simulink model "FullED"  (R2023b)
settings: Solver=VariableStepAuto  StartTime=0.0  StopTime=3000/fs  RelTol=1e-3
undefined symbols (not defined in the file): exp_W1, exp_W2, exp_W3, exp_W4, fs
libraries: hdlBasic x155, hdlDSPIP x8, hdlsllib x2, vmcUtilities x1
(part 1 of 2)
settings Model: Creator=jojok  LastModifiedBy=jojok

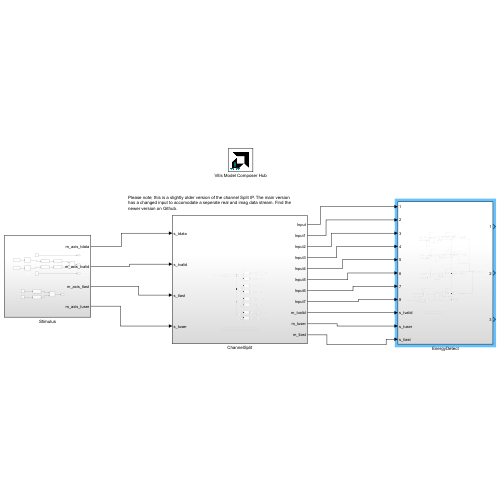
[thumbnail: Simulink's stored preview of the top-level diagram]
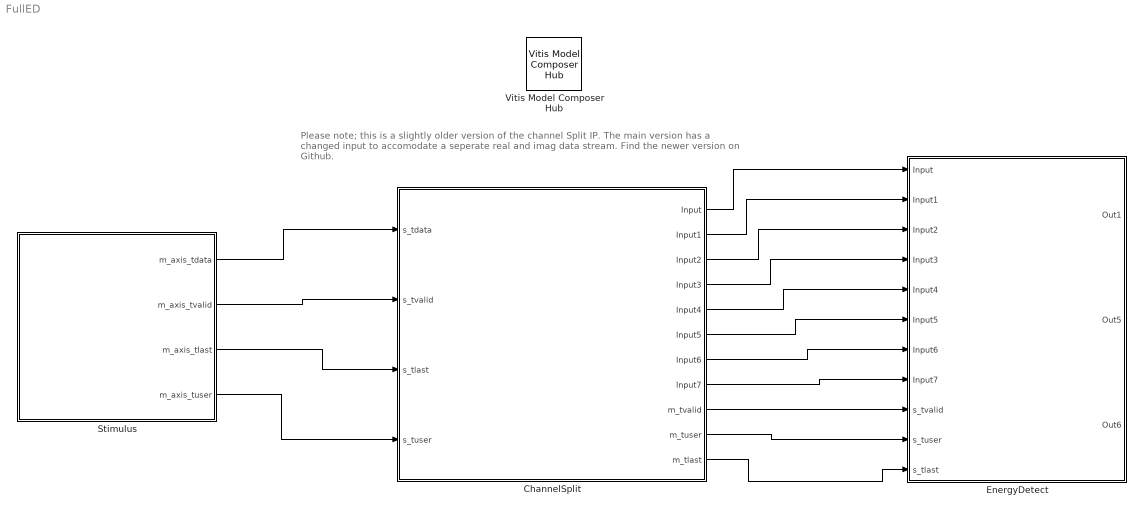
== system FullED ==
  note: Please note; this is a slightly older version of the channel Split IP. The main version
      | has a changed input to accomodate a seperate real and imag data stream. Find the newer version on Github.
  ChannelSplit : Subsystem
  EnergyDetect : Subsystem
  Stimulus : Subsystem
  Vitis Model Composer Hub : vmcUtilities/Vitis Model Composer Hub  Tag=genX  CodeGeneration=off  SubsystemName=ChannelSplit  DUTSubsystemName=EnergyDetect  CompilationType=HDLCompilation  ExportTypeV2=IP Catalog  TargetDirectory=./netlistFullED\ip\EnergyDetect\src  exportDesign=on  analyzeDesign=off  validateDesignOnHw=off  ExportType=HDL  IpVendor=xilinx.com  IpLibrary=hls  IpVersion=1.0  IpHWLanguage=Verilog  AieCompilerOptions={}  AieSimulatorOptions={}  CreateTestbench=off  TestbenchStackSize=10  RunRtlSim=off  RunCSim=off  RunAieSim=off  AieSimTimeout=50000  RunAieSimProfiling=off  LaunchVitisAnalyzer=off  PlotOutput=off  RunX86Sim=off  X86SimTimeout=10  GenHwImage=off  GenLibadfXo=on  GenHwValidationCode=off  PlatformType=Not Specified  HwSystemType=Baremetal  HwValidationTarget=hw  ProjDevice=xczu28dr-ffvg1517-2-e  ProjDevicePart=xczu28dr-ffvg1517-2-e  SamplePeriod=-1  ClockFrequency=200  DataPathParallelism=1  xilinxfamily=zynquplusRFSOC  part=xczu28dr  speed=-2-e  package=ffvg1517  directory=./netlist\ip\ChannelSplit\src  testbench=off  incr_netlist=off  synthesis_tool=Vivado  clock_wrapper=Clock Enables  dbl_ovrd=According to Block Masks  dcm_input_clock_period=10  sysclk_period=(1/fs)*(1e6)  simulink_period=1/(51200000)  eval_field=0  IPInfoJsonString="{\"HDLSubsystem\":{\"SubsystemName\":\"EnergyDetect\",\"IPName\":\"EnergyDetect\",\"IPLibrary\":\"VMC\",\"IPVendor\":\"CoRSoC\",\"IPVersion\":\"1.1\",\"TargetDirectory\":\"./netlistFullED\",\"SubsystemDir\":\"./netlistFullED\\\\ip\\\\EnergyDetect\"},\"SubsystemTag\":\"HDLNode\"}"  LogFileName=''  NThreads=4
  wires:
  Stimulus/1(m_axis_tdata) -> ChannelSplit/1(s_tdata)
  Stimulus/2(m_axis_tvalid) -> ChannelSplit/2(s_tvalid)
  Stimulus/3(m_axis_tlast) -> ChannelSplit/3(s_tlast)
  ChannelSplit/11(m_tlast) -> EnergyDetect/11(s_tlast)
  ChannelSplit/9(m_tvalid) -> EnergyDetect/9(s_tvalid)
  ChannelSplit/8(Input7) -> EnergyDetect/8(Input7)
  ChannelSplit/7(Input6) -> EnergyDetect/7(Input6)
  ChannelSplit/6(Input5) -> EnergyDetect/6(Input5)
  ChannelSplit/5(Input4) -> EnergyDetect/5(Input4)
  ChannelSplit/4(Input3) -> EnergyDetect/4(Input3)
  ChannelSplit/3(Input2) -> EnergyDetect/3(Input2)
  ChannelSplit/2(Input1) -> EnergyDetect/2(Input1)
  ChannelSplit/1(Input) -> EnergyDetect/1(Input)
  Stimulus/4(m_axis_tuser) -> ChannelSplit/4(s_tuser)
  ChannelSplit/10(m_tuser) -> EnergyDetect/10(s_tuser)

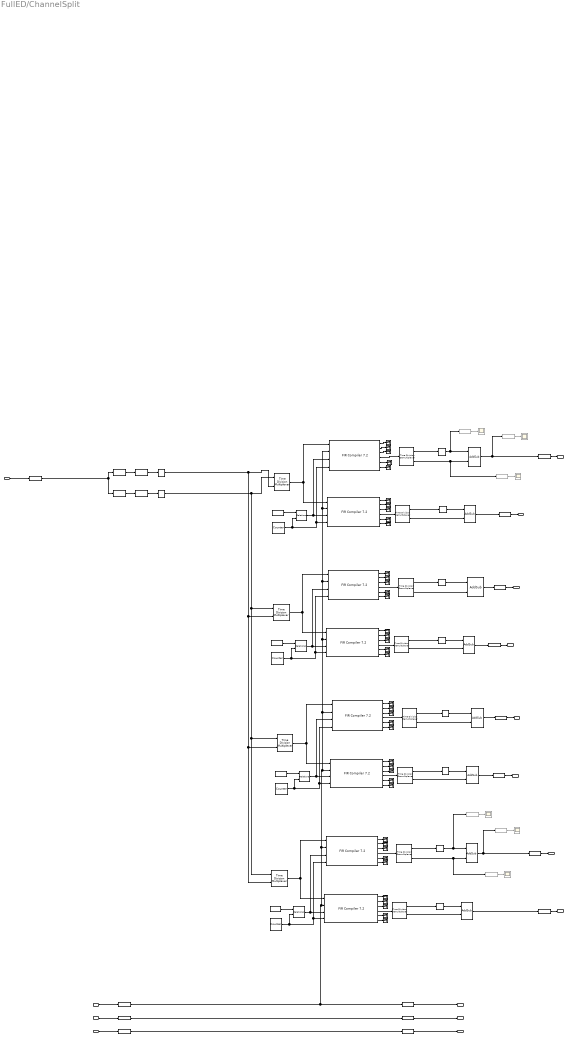
== system FullED/ChannelSplit ==
  note: https://x.com/ChineseEmbinUS/status/1909350269009219937
  note: a[n]
  note: Split the signal into real and imaginary components
  note: b[n]
  note: a[n]
  note: b[n]
  note: a[n]
  note: b[n]
  note: a[n]
  note: b[n]
  s_tdata : Inport
  s_tvalid : Inport  Port=2
  s_tlast : Inport  Port=3
  s_tuser : Inport  Port=4
  AddSub{,2,4,6} (4 alike) : hdlBasic/AddSub  mode=Subtraction  use_carryin=off  use_carryout=off  en=off  latency=1  precision=Full  arith_type=Unsigned  n_bits=16  bin_pt=14  quantization=Truncate  overflow=Wrap  use_behavioral_HDL=off  hw_selection=Fabric  pipelined=off  XmcBlockStatus=1  maskContainerNames=tabcontainer1  block_type=addsub  block_config=sysgen:Addsub_config
  AddSub{1,3,5,7} (4 alike) : hdlBasic/AddSub  mode=Addition  use_carryin=off  use_carryout=off  en=off  latency=1  precision=Full  arith_type=Unsigned  n_bits=16  bin_pt=14  quantization=Truncate  overflow=Wrap  use_behavioral_HDL=off  hw_selection=Fabric  pipelined=off  XmcBlockStatus=1  maskContainerNames=tabcontainer1  block_type=addsub  block_config=sysgen:Addsub_config
  Constant{5,8,12,16} (4 alike) : hdlBasic/Constant  const=1.0  gui_display_data_type=Fixed-point  arith_type=Signed (2's comp)  n_bits=16  bin_pt=14  preci_type=Single  exp_width=8  frac_width=24  explicit_period=off  period=1  XmcBlockStatus=1  maskContainerNames=tabcontainer1  block_type=constant  block_config=sysgen:Constant_config
  Counter{,2,4,6} (4 alike) : hdlBasic/Counter  cnt_type=Count limited  cnt_to=1  operation=Up  start_count=0  cnt_by_val=1  arith_type=Unsigned  n_bits=1  bin_pt=0  load_pin=off  rst=off  en=off  explicit_period=Explicit  period=1/(2*fs)  use_behavioral_HDL=off  implementation=Fabric  XmcBlockStatus=1  maskContainerNames=group1  block_type=counter  block_config=sysgen:Counter_config  block_width=531  block_height=1023
  Delay{1,3..4,8..9,11..12,15..16,20} (10 alike) : hdlBasic/Delay  rst=off  en=off  latency=1  reg_retiming=off  XmcBlockStatus=1  maskContainerNames=group1  block_type=delay  block_config=sysgen:Delay_config
  FIR Compiler 7.1 : hdlDSPIP/FIR Compiler 7.2   coefficientvector=[real(exp_W1), imag(exp_W1)]  coefficient_sets=2  coefficient_reload=off  filter_type=Single_Rate  rate_change_type=Integer  interpolation_rate=1  decimation_rate=1  zero_pack_factor=1  channel_sequence=Basic  number_channels=2  pattern_list='P4-0,P4-1,P4-2,P4-3,P4-4'  number_paths=1  ratespecification=Maximum_Possible  sampleperiod=1  hardwareoversamplingrate=1  coefficient_sign=Signed  quantization=Quantize_Only  coefficient_width=16  bestprecision=off  coefficient_fractional_bits=15  coefficient_structure=Inferred  output_rounding_mode=Full_Precision  output_width=32  filter_architecture=Systolic_Multiply_Accumulate  optimization_goal=Area  optimization_list='None'  data_buffer_type=Automatic  coefficient_buffer_type=Automatic  input_buffer_type=Automatic  output_buffer_type=Automatic  preference_for_other_storage=Automatic  multi_column_support=Automatic  columnconfig='117'  inter_column_pipe_length=4  data_has_tlast=Not_Required  m_data_has_tready=off  s_data_has_fifo=off  s_data_has_tuser=Not_Required  m_data_has_tuser=Not_Required  s_config_sync_mode=On_Vector  s_config_method=By_Channel  num_reload_slots=1  has_aclken=off  has_aresetn=off  reset_data_vector=on  trim_axipin_name=on  simulation_type=hybrid_sim  simulation_model=sysgen:xfirv7_2_cmodel  data_path_portlist={ 's_axis_data_tdata', 'm_axis_data_tdata' }  passband_min=0.0  passband_max=0.5  stopband_min=0.5  stopband_max=1.0  filter_selection=1  gui_behaviour='Sysgen_GUI'  data_sign=Signed  data_width=16  data_fractional_bits=0  data_tuser_width=1  wrapper_available=true  ip_wrap_arbitrary_binary_point=true  ip_name=FIR Compiler  ip_version=7.2  dsptool_ready=true  ipcore_usecache=true  ipcore_useipmodelcache=true  port_translation_map={ 'aclken' => 'en', 'aresetn' => 'rst' }  run_core_at_system_period=true  ipcore_xco_need_fpga_part=true  ipcore_fpga_part=[]  XmcBlockStatus=1  maskContainerNames=tabcontainer1  block_type=fir_compiler_v7_2  block_config=sysgen:rodinimport_config  block_width=820  block_height=600
  FIR Compiler 7.2 : hdlDSPIP/FIR Compiler 7.2   coefficientvector=[imag(exp_W1), real(exp_W1)]  coefficient_sets=2  coefficient_reload=off  filter_type=Single_Rate  rate_change_type=Integer  interpolation_rate=1  decimation_rate=1  zero_pack_factor=1  channel_sequence=Basic  number_channels=2  pattern_list='P4-0,P4-1,P4-2,P4-3,P4-4'  number_paths=1  ratespecification=Maximum_Possible  sampleperiod=1  hardwareoversamplingrate=1  coefficient_sign=Signed  quantization=Quantize_Only  coefficient_width=16  bestprecision=off  coefficient_fractional_bits=15  coefficient_structure=Inferred  output_rounding_mode=Full_Precision  output_width=32  filter_architecture=Systolic_Multiply_Accumulate  optimization_goal=Area  optimization_list='None'  data_buffer_type=Automatic  coefficient_buffer_type=Automatic  input_buffer_type=Automatic  output_buffer_type=Automatic  preference_for_other_storage=Automatic  multi_column_support=Automatic  columnconfig='117'  inter_column_pipe_length=4  data_has_tlast=Not_Required  m_data_has_tready=off  s_data_has_fifo=off  s_data_has_tuser=Not_Required  m_data_has_tuser=Not_Required  s_config_sync_mode=On_Vector  s_config_method=By_Channel  num_reload_slots=1  has_aclken=off  has_aresetn=off  reset_data_vector=on  trim_axipin_name=on  simulation_type=hybrid_sim  simulation_model=sysgen:xfirv7_2_cmodel  data_path_portlist={ 's_axis_data_tdata', 'm_axis_data_tdata' }  passband_min=0.0  passband_max=0.5  stopband_min=0.5  stopband_max=1.0  filter_selection=1  gui_behaviour='Sysgen_GUI'  data_sign=Signed  data_width=16  data_fractional_bits=0  data_tuser_width=1  wrapper_available=true  ip_wrap_arbitrary_binary_point=true  ip_name=FIR Compiler  ip_version=7.2  dsptool_ready=true  ipcore_usecache=true  ipcore_useipmodelcache=true  port_translation_map={ 'aclken' => 'en', 'aresetn' => 'rst' }  run_core_at_system_period=true  ipcore_xco_need_fpga_part=true  ipcore_fpga_part=[]  XmcBlockStatus=1  maskContainerNames=tabcontainer1  block_type=fir_compiler_v7_2  block_config=sysgen:rodinimport_config  block_width=820  block_height=600
  FIR Compiler 7.3 : hdlDSPIP/FIR Compiler 7.2   coefficientvector=[real(exp_W2), imag(exp_W2)]  coefficient_sets=2  coefficient_reload=off  filter_type=Single_Rate  rate_change_type=Integer  interpolation_rate=1  decimation_rate=1  zero_pack_factor=1  channel_sequence=Basic  number_channels=2  pattern_list='P4-0,P4-1,P4-2,P4-3,P4-4'  number_paths=1  ratespecification=Maximum_Possible  sampleperiod=1  hardwareoversamplingrate=1  coefficient_sign=Signed  quantization=Quantize_Only  coefficient_width=16  bestprecision=off  coefficient_fractional_bits=15  coefficient_structure=Inferred  output_rounding_mode=Full_Precision  output_width=32  filter_architecture=Systolic_Multiply_Accumulate  optimization_goal=Area  optimization_list='None'  data_buffer_type=Automatic  coefficient_buffer_type=Automatic  input_buffer_type=Automatic  output_buffer_type=Automatic  preference_for_other_storage=Automatic  multi_column_support=Automatic  columnconfig='117'  inter_column_pipe_length=4  data_has_tlast=Not_Required  m_data_has_tready=off  s_data_has_fifo=off  s_data_has_tuser=Not_Required  m_data_has_tuser=Not_Required  s_config_sync_mode=On_Vector  s_config_method=By_Channel  num_reload_slots=1  has_aclken=off  has_aresetn=off  reset_data_vector=on  trim_axipin_name=on  simulation_type=hybrid_sim  simulation_model=sysgen:xfirv7_2_cmodel  data_path_portlist={ 's_axis_data_tdata', 'm_axis_data_tdata' }  passband_min=0.0  passband_max=0.5  stopband_min=0.5  stopband_max=1.0  filter_selection=1  gui_behaviour='Sysgen_GUI'  data_sign=Signed  data_width=16  data_fractional_bits=0  data_tuser_width=1  wrapper_available=true  ip_wrap_arbitrary_binary_point=true  ip_name=FIR Compiler  ip_version=7.2  dsptool_ready=true  ipcore_usecache=true  ipcore_useipmodelcache=true  port_translation_map={ 'aclken' => 'en', 'aresetn' => 'rst' }  run_core_at_system_period=true  ipcore_xco_need_fpga_part=true  ipcore_fpga_part=[]  XmcBlockStatus=1  maskContainerNames=tabcontainer1  block_type=fir_compiler_v7_2  block_config=sysgen:rodinimport_config  block_width=820  block_height=600
  FIR Compiler 7.4 : hdlDSPIP/FIR Compiler 7.2   coefficientvector=[imag(exp_W2), real(exp_W2)]  coefficient_sets=2  coefficient_reload=off  filter_type=Single_Rate  rate_change_type=Integer  interpolation_rate=1  decimation_rate=1  zero_pack_factor=1  channel_sequence=Basic  number_channels=2  pattern_list='P4-0,P4-1,P4-2,P4-3,P4-4'  number_paths=1  ratespecification=Maximum_Possible  sampleperiod=1  hardwareoversamplingrate=1  coefficient_sign=Signed  quantization=Quantize_Only  coefficient_width=16  bestprecision=off  coefficient_fractional_bits=15  coefficient_structure=Inferred  output_rounding_mode=Full_Precision  output_width=32  filter_architecture=Systolic_Multiply_Accumulate  optimization_goal=Area  optimization_list='None'  data_buffer_type=Automatic  coefficient_buffer_type=Automatic  input_buffer_type=Automatic  output_buffer_type=Automatic  preference_for_other_storage=Automatic  multi_column_support=Automatic  columnconfig='117'  inter_column_pipe_length=4  data_has_tlast=Not_Required  m_data_has_tready=off  s_data_has_fifo=off  s_data_has_tuser=Not_Required  m_data_has_tuser=Not_Required  s_config_sync_mode=On_Vector  s_config_method=By_Channel  num_reload_slots=1  has_aclken=off  has_aresetn=off  reset_data_vector=on  trim_axipin_name=on  simulation_type=hybrid_sim  simulation_model=sysgen:xfirv7_2_cmodel  data_path_portlist={ 's_axis_data_tdata', 'm_axis_data_tdata' }  passband_min=0.0  passband_max=0.5  stopband_min=0.5  stopband_max=1.0  filter_selection=1  gui_behaviour='Sysgen_GUI'  data_sign=Signed  data_width=16  data_fractional_bits=0  data_tuser_width=1  wrapper_available=true  ip_wrap_arbitrary_binary_point=true  ip_name=FIR Compiler  ip_version=7.2  dsptool_ready=true  ipcore_usecache=true  ipcore_useipmodelcache=true  port_translation_map={ 'aclken' => 'en', 'aresetn' => 'rst' }  run_core_at_system_period=true  ipcore_xco_need_fpga_part=true  ipcore_fpga_part=[]  XmcBlockStatus=1  maskContainerNames=tabcontainer1  block_type=fir_compiler_v7_2  block_config=sysgen:rodinimport_config  block_width=820  block_height=600
  FIR Compiler 7.5 : hdlDSPIP/FIR Compiler 7.2   coefficientvector=[real(exp_W3), imag(exp_W3)]  coefficient_sets=2  coefficient_reload=off  filter_type=Single_Rate  rate_change_type=Integer  interpolation_rate=1  decimation_rate=1  zero_pack_factor=1  channel_sequence=Basic  number_channels=2  pattern_list='P4-0,P4-1,P4-2,P4-3,P4-4'  number_paths=1  ratespecification=Maximum_Possible  sampleperiod=1  hardwareoversamplingrate=1  coefficient_sign=Signed  quantization=Quantize_Only  coefficient_width=16  bestprecision=off  coefficient_fractional_bits=15  coefficient_structure=Inferred  output_rounding_mode=Full_Precision  output_width=32  filter_architecture=Systolic_Multiply_Accumulate  optimization_goal=Area  optimization_list='None'  data_buffer_type=Automatic  coefficient_buffer_type=Automatic  input_buffer_type=Automatic  output_buffer_type=Automatic  preference_for_other_storage=Automatic  multi_column_support=Automatic  columnconfig='117'  inter_column_pipe_length=4  data_has_tlast=Not_Required  m_data_has_tready=off  s_data_has_fifo=off  s_data_has_tuser=Not_Required  m_data_has_tuser=Not_Required  s_config_sync_mode=On_Vector  s_config_method=By_Channel  num_reload_slots=1  has_aclken=off  has_aresetn=off  reset_data_vector=on  trim_axipin_name=on  simulation_type=hybrid_sim  simulation_model=sysgen:xfirv7_2_cmodel  data_path_portlist={ 's_axis_data_tdata', 'm_axis_data_tdata' }  passband_min=0.0  passband_max=0.5  stopband_min=0.5  stopband_max=1.0  filter_selection=1  gui_behaviour='Sysgen_GUI'  data_sign=Signed  data_width=16  data_fractional_bits=0  data_tuser_width=1  wrapper_available=true  ip_wrap_arbitrary_binary_point=true  ip_name=FIR Compiler  ip_version=7.2  dsptool_ready=true  ipcore_usecache=true  ipcore_useipmodelcache=true  port_translation_map={ 'aclken' => 'en', 'aresetn' => 'rst' }  run_core_at_system_period=true  ipcore_xco_need_fpga_part=true  ipcore_fpga_part=[]  XmcBlockStatus=1  maskContainerNames=tabcontainer1  block_type=fir_compiler_v7_2  block_config=sysgen:rodinimport_config  block_width=820  block_height=600
  FIR Compiler 7.6 : hdlDSPIP/FIR Compiler 7.2   coefficientvector=[imag(exp_W3), real(exp_W3)]  coefficient_sets=2  coefficient_reload=off  filter_type=Single_Rate  rate_change_type=Integer  interpolation_rate=1  decimation_rate=1  zero_pack_factor=1  channel_sequence=Basic  number_channels=2  pattern_list='P4-0,P4-1,P4-2,P4-3,P4-4'  number_paths=1  ratespecification=Maximum_Possible  sampleperiod=1  hardwareoversamplingrate=1  coefficient_sign=Signed  quantization=Quantize_Only  coefficient_width=16  bestprecision=off  coefficient_fractional_bits=15  coefficient_structure=Inferred  output_rounding_mode=Full_Precision  output_width=32  filter_architecture=Systolic_Multiply_Accumulate  optimization_goal=Area  optimization_list='None'  data_buffer_type=Automatic  coefficient_buffer_type=Automatic  input_buffer_type=Automatic  output_buffer_type=Automatic  preference_for_other_storage=Automatic  multi_column_support=Automatic  columnconfig='117'  inter_column_pipe_length=4  data_has_tlast=Not_Required  m_data_has_tready=off  s_data_has_fifo=off  s_data_has_tuser=Not_Required  m_data_has_tuser=Not_Required  s_config_sync_mode=On_Vector  s_config_method=By_Channel  num_reload_slots=1  has_aclken=off  has_aresetn=off  reset_data_vector=on  trim_axipin_name=on  simulation_type=hybrid_sim  simulation_model=sysgen:xfirv7_2_cmodel  data_path_portlist={ 's_axis_data_tdata', 'm_axis_data_tdata' }  passband_min=0.0  passband_max=0.5  stopband_min=0.5  stopband_max=1.0  filter_selection=1  gui_behaviour='Sysgen_GUI'  data_sign=Signed  data_width=16  data_fractional_bits=0  data_tuser_width=1  wrapper_available=true  ip_wrap_arbitrary_binary_point=true  ip_name=FIR Compiler  ip_version=7.2  dsptool_ready=true  ipcore_usecache=true  ipcore_useipmodelcache=true  port_translation_map={ 'aclken' => 'en', 'aresetn' => 'rst' }  run_core_at_system_period=true  ipcore_xco_need_fpga_part=true  ipcore_fpga_part=[]  XmcBlockStatus=1  maskContainerNames=tabcontainer1  block_type=fir_compiler_v7_2  block_config=sysgen:rodinimport_config  block_width=820  block_height=600
  FIR Compiler 7.7 : hdlDSPIP/FIR Compiler 7.2   coefficientvector=[real(exp_W4), imag(exp_W4)]  coefficient_sets=2  coefficient_reload=off  filter_type=Single_Rate  rate_change_type=Integer  interpolation_rate=1  decimation_rate=1  zero_pack_factor=1  channel_sequence=Basic  number_channels=2  pattern_list='P4-0,P4-1,P4-2,P4-3,P4-4'  number_paths=1  ratespecification=Maximum_Possible  sampleperiod=1  hardwareoversamplingrate=1  coefficient_sign=Signed  quantization=Quantize_Only  coefficient_width=16  bestprecision=off  coefficient_fractional_bits=15  coefficient_structure=Inferred  output_rounding_mode=Full_Precision  output_width=32  filter_architecture=Systolic_Multiply_Accumulate  optimization_goal=Area  optimization_list='None'  data_buffer_type=Automatic  coefficient_buffer_type=Automatic  input_buffer_type=Automatic  output_buffer_type=Automatic  preference_for_other_storage=Automatic  multi_column_support=Automatic  columnconfig='117'  inter_column_pipe_length=4  data_has_tlast=Not_Required  m_data_has_tready=off  s_data_has_fifo=off  s_data_has_tuser=Not_Required  m_data_has_tuser=Not_Required  s_config_sync_mode=On_Vector  s_config_method=By_Channel  num_reload_slots=1  has_aclken=off  has_aresetn=off  reset_data_vector=on  trim_axipin_name=on  simulation_type=hybrid_sim  simulation_model=sysgen:xfirv7_2_cmodel  data_path_portlist={ 's_axis_data_tdata', 'm_axis_data_tdata' }  passband_min=0.0  passband_max=0.5  stopband_min=0.5  stopband_max=1.0  filter_selection=1  gui_behaviour='Sysgen_GUI'  data_sign=Signed  data_width=16  data_fractional_bits=0  data_tuser_width=1  wrapper_available=true  ip_wrap_arbitrary_binary_point=true  ip_name=FIR Compiler  ip_version=7.2  dsptool_ready=true  ipcore_usecache=true  ipcore_useipmodelcache=true  port_translation_map={ 'aclken' => 'en', 'aresetn' => 'rst' }  run_core_at_system_period=true  ipcore_xco_need_fpga_part=true  ipcore_fpga_part=[]  XmcBlockStatus=1  maskContainerNames=tabcontainer1  block_type=fir_compiler_v7_2  block_config=sysgen:rodinimport_config  block_width=820  block_height=600
  FIR Compiler 7.8 : hdlDSPIP/FIR Compiler 7.2   coefficientvector=[imag(exp_W4), real(exp_W4)]  coefficient_sets=2  coefficient_reload=off  filter_type=Single_Rate  rate_change_type=Integer  interpolation_rate=1  decimation_rate=1  zero_pack_factor=1  channel_sequence=Basic  number_channels=2  pattern_list='P4-0,P4-1,P4-2,P4-3,P4-4'  number_paths=1  ratespecification=Maximum_Possible  sampleperiod=1  hardwareoversamplingrate=1  coefficient_sign=Signed  quantization=Quantize_Only  coefficient_width=16  bestprecision=off  coefficient_fractional_bits=15  coefficient_structure=Inferred  output_rounding_mode=Full_Precision  output_width=32  filter_architecture=Systolic_Multiply_Accumulate  optimization_goal=Area  optimization_list='None'  data_buffer_type=Automatic  coefficient_buffer_type=Automatic  input_buffer_type=Automatic  output_buffer_type=Automatic  preference_for_other_storage=Automatic  multi_column_support=Automatic  columnconfig='117'  inter_column_pipe_length=4  data_has_tlast=Not_Required  m_data_has_tready=off  s_data_has_fifo=off  s_data_has_tuser=Not_Required  m_data_has_tuser=Not_Required  s_config_sync_mode=On_Vector  s_config_method=By_Channel  num_reload_slots=1  has_aclken=off  has_aresetn=off  reset_data_vector=on  trim_axipin_name=on  simulation_type=hybrid_sim  simulation_model=sysgen:xfirv7_2_cmodel  data_path_portlist={ 's_axis_data_tdata', 'm_axis_data_tdata' }  passband_min=0.0  passband_max=0.5  stopband_min=0.5  stopband_max=1.0  filter_selection=1  gui_behaviour='Sysgen_GUI'  data_sign=Signed  data_width=16  data_fractional_bits=0  data_tuser_width=1  wrapper_available=true  ip_wrap_arbitrary_binary_point=true  ip_name=FIR Compiler  ip_version=7.2  dsptool_ready=true  ipcore_usecache=true  ipcore_useipmodelcache=true  port_translation_map={ 'aclken' => 'en', 'aresetn' => 'rst' }  run_core_at_system_period=true  ipcore_xco_need_fpga_part=true  ipcore_fpga_part=[]  XmcBlockStatus=1  maskContainerNames=tabcontainer1  block_type=fir_compiler_v7_2  block_config=sysgen:rodinimport_config  block_width=820  block_height=600
  Gateway Out{2..4,6..8} (6 alike) : hdlBasic/Gateway Out  Commented=on  inherit_from_input=off  hdl_port=off  rows=1  columns=1  UseAsDAC=off  DACChannel='1'  interface=None  automatic_assignment=on  address_offset=hex2dec('00')  intf_name=''  intf_description=''  timing_constraint=None  locs_specified=off  LOCs={}  io_standard={}  XmcBlockStatus=1  maskContainerNames=group4  block_type=gatewayout  block_config=sysgen:gateway_out_config  block_width_w=590  block_height_w=620  block_width=620  block_height=750
  Imaginary1 : hdlBasic/Slice  nbits=16  boolean_output=off  mode=Two Bit Locations  bit1=31  base1=LSB of Input  bit0=16  base0=LSB of Input  XmcBlockStatus=1  maskContainerNames=group1  block_type=slice  block_config=sysgen:Slice_config
  Real1 : hdlBasic/Slice  nbits=16  boolean_output=off  mode=Two Bit Locations  bit1=15  base1=LSB of Input  bit0=0  base0=LSB of Input  XmcBlockStatus=1  maskContainerNames=group1  block_type=slice  block_config=sysgen:Slice_config
  Reinterpret1 : hdlBasic/Reinterpret  force_arith_type=on  arith_type="Signed  (2's comp)"  force_bin_pt=on  bin_pt=14  XmcBlockStatus=1  maskContainerNames=group1  block_type=reinterpret  block_config=sysgen:Reinterpret_config
  Reinterpret7 : hdlBasic/Reinterpret  force_arith_type=on  arith_type="Signed  (2's comp)"  force_bin_pt=on  bin_pt=14  XmcBlockStatus=1  maskContainerNames=group1  block_type=reinterpret  block_config=sysgen:Reinterpret_config
  Relational{1,4,7,10} (4 alike) : hdlBasic/Relational  mode=a=b  op_type=Bool  en=off  latency=1  XmcBlockStatus=1  maskContainerNames=tabcontainer1  block_type=relational  block_config=sysgen:Relational_config
  Terminator{1..8,10..21,23..32,34..43} (40 alike) : Terminator
  Time Scope{3..4,6..8} (5 alike) : Scope  Commented=on
  Time ScopeTwo : Scope  Commented=on
  Time Division Demultiplexer{,1..7} (8 alike) : hdlBasic/Time Division Demultiplexer  frame_pattern=[1 1]  impl_style=Multiple Channel  vin=off  explicit_period=off  period=1  XmcBlockStatus=1  maskContainerNames=group2  block_type=tdd  block_config=sysgen:TDD_config
  Time Division Multiplexer{,1..3} (4 alike) : hdlBasic/Time Division Multiplexer  inputs=2  vin=off  Optimization=Resource  explicit_period=off  period=1  XmcBlockStatus=1  maskContainerNames=group3  block_type=tdm  block_config=sysgen:TDM_config
  m_axis_tdata{1..8} (8 alike) : hdlBasic/Gateway Out  inherit_from_input=on  hdl_port=on  rows=1  columns=1  UseAsDAC=off  DACChannel='1'  interface=None  automatic_assignment=on  address_offset=hex2dec('00')  intf_name=''  intf_description=''  timing_constraint=None  locs_specified=off  LOCs={}  io_standard={}  XmcBlockStatus=1  maskContainerNames=group4  block_type=gatewayout  block_config=sysgen:gateway_out_config  block_width_w=590  block_height_w=620  block_width=620  block_height=750
  m_axis_tlast : hdlBasic/Gateway Out  inherit_from_input=on  hdl_port=on  rows=1  columns=1  UseAsDAC=off  DACChannel='1'  interface=None  automatic_assignment=on  address_offset=hex2dec('00')  intf_name=''  intf_description=''  timing_constraint=None  locs_specified=off  LOCs={}  io_standard={}  XmcBlockStatus=1  maskContainerNames=group4  block_type=gatewayout  block_config=sysgen:gateway_out_config  block_width_w=590  block_height_w=620  block_width=620  block_height=750
  m_axis_tuser : hdlBasic/Gateway Out  inherit_from_input=on  hdl_port=on  rows=1  columns=1  UseAsDAC=off  DACChannel='1'  interface=None  automatic_assignment=on  address_offset=hex2dec('00')  intf_name=''  intf_description=''  timing_constraint=None  locs_specified=off  LOCs={}  io_standard={}  XmcBlockStatus=1  maskContainerNames=group4  block_type=gatewayout  block_config=sysgen:gateway_out_config  block_width_w=590  block_height_w=620  block_width=620  block_height=750
  m_axis_tvalid : hdlBasic/Gateway Out  inherit_from_input=on  hdl_port=on  rows=1  columns=1  UseAsDAC=off  DACChannel='1'  interface=None  automatic_assignment=on  address_offset=hex2dec('00')  intf_name=''  intf_description=''  timing_constraint=None  locs_specified=off  LOCs={}  io_standard={}  XmcBlockStatus=1  maskContainerNames=group4  block_type=gatewayout  block_config=sysgen:gateway_out_config  block_width_w=590  block_height_w=620  block_width=620  block_height=750
  s_axis_tdata : hdlBasic/Gateway In  gui_display_data_type=Fixed-point  arith_type=Unsigned  n_bits=32  bin_pt=0  preci_type=Single  exp_width=8  frac_width=24  rows=1  columns=1  quantization="Round  (unbiased: +/- Inf)"  overflow=Saturate  period=1/fs  UseAsADC=off  ADCChannel='1'  interface=None  automatic_assignment=on  address_offset=hex2dec('00')  intf_name=''  intf_description=''  default_value=0  timing_constraint=None  locs_specified=off  LOCs={}  io_standard={}  inherit_from_input=off  hdl_port=on  XmcBlockStatus=1  maskContainerNames=group4  block_type=gatewayin  block_config=sysgen:gateway_in_config  block_width_w=590  block_height_w=620  block_width=640  block_height=850
  s_axis_tlast : hdlBasic/Gateway In  gui_display_data_type=Boolean  arith_type=Boolean  n_bits=16  bin_pt=14  preci_type=Single  exp_width=8  frac_width=24  rows=1  columns=1  quantization="Round  (unbiased: +/- Inf)"  overflow=Saturate  period=1/fs  UseAsADC=off  ADCChannel='1'  interface=None  automatic_assignment=on  address_offset=hex2dec('00')  intf_name=''  intf_description=''  default_value=0  timing_constraint=None  locs_specified=off  LOCs={}  io_standard={}  inherit_from_input=off  hdl_port=on  XmcBlockStatus=1  maskContainerNames=group4  block_type=gatewayin  block_config=sysgen:gateway_in_config  block_width_w=590  block_height_w=620  block_width=640  block_height=850
  s_axis_tuser : hdlBasic/Gateway In  gui_display_data_type=Fixed-point  arith_type=Signed (2's comp)  n_bits=32  bin_pt=0  preci_type=Single  exp_width=8  frac_width=24  rows=1  columns=1  quantization="Round  (unbiased: +/- Inf)"  overflow=Saturate  period=1/fs  UseAsADC=off  ADCChannel='1'  interface=None  automatic_assignment=on  address_offset=hex2dec('00')  intf_name=''  intf_description=''  default_value=0  timing_constraint=None  locs_specified=off  LOCs={}  io_standard={}  inherit_from_input=off  hdl_port=on  XmcBlockStatus=1  maskContainerNames=group4  block_type=gatewayin  block_config=sysgen:gateway_in_config  block_width_w=590  block_height_w=620  block_width=640  block_height=850
  s_axis_tvalid : hdlBasic/Gateway In  gui_display_data_type=Boolean  arith_type=Boolean  n_bits=16  bin_pt=14  preci_type=Single  exp_width=8  frac_width=24  rows=1  columns=1  quantization="Round  (unbiased: +/- Inf)"  overflow=Saturate  period=1/fs  UseAsADC=off  ADCChannel='1'  interface=None  automatic_assignment=on  address_offset=hex2dec('00')  intf_name=''  intf_description=''  default_value=0  timing_constraint=None  locs_specified=off  LOCs={}  io_standard={}  inherit_from_input=off  hdl_port=on  XmcBlockStatus=1  maskContainerNames=group4  block_type=gatewayin  block_config=sysgen:gateway_in_config  block_width_w=590  block_height_w=620  block_width=640  block_height=850
  Input : Outport
  Input1 : Outport  Port=2
  Input2 : Outport  Port=3
  Input3 : Outport  Port=4
  Input4 : Outport  Port=5
  Input5 : Outport  Port=6
  Input6 : Outport  Port=7
  Input7 : Outport  Port=8
  m_tvalid : Outport  Port=9
  m_tuser : Outport  Port=10
  m_tlast : Outport  Port=11
  wires:
  FIR Compiler 7.1/3 -> Terminator3/1
  FIR Compiler 7.2/5 -> Terminator11/1
  FIR Compiler 7.1/2 -> Terminator4/1
  FIR Compiler 7.1/6 -> Terminator1/1
  Delay11/1 -> Time Division Multiplexer3/1, Time Division Multiplexer2/1, Time Division Multiplexer1/1, Time Division Multiplexer/1
  Delay3/1 -> AddSub1/1
  Time Division Demultiplexer1/2 -> AddSub1/2
  Counter/1 -> FIR Compiler 7.2/4, FIR Compiler 7.1/4, Relational1/2
  Reinterpret1/1 -> Delay12/1
  FIR Compiler 7.2/2 -> Terminator7/1
  Real1/1 -> Reinterpret7/1
  s_axis_tdata/1 -> Real1/1, Imaginary1/1
  FIR Compiler 7.2/3 -> Terminator8/1
  Constant5/1 -> Relational1/1
  FIR Compiler 7.1/4 -> Time Division Demultiplexer/1
  s_tdata/1 -> s_axis_tdata/1
  Reinterpret7/1 -> Delay11/1
  FIR Compiler 7.2/1 -> Terminator6/1
  Time Division Demultiplexer1/1 -> Delay3/1
  FIR Compiler 7.1/1 -> Terminator5/1
  FIR Compiler 7.2/6 -> Terminator12/1
  Imaginary1/1 -> Reinterpret1/1
  Time Division Multiplexer/1 -> FIR Compiler 7.2/1, FIR Compiler 7.1/1
  FIR Compiler 7.1/5 -> Terminator2/1
  FIR Compiler 7.2/4 -> Time Division Demultiplexer1/1
  Relational1/1 -> FIR Compiler 7.2/3, FIR Compiler 7.1/3
  Delay12/1 -> Time Division Multiplexer3/2, Time Division Multiplexer2/2, Time Division Multiplexer1/2, Time Division Multiplexer/2
  Constant8/1 -> Relational4/1
  FIR Compiler 7.4/3 -> Terminator21/1
  FIR Compiler 7.3/4 -> Time Division Demultiplexer2/1
  Time Division Demultiplexer2/1 -> Delay4/1
  FIR Compiler 7.4/6 -> Terminator14/1
  Time Division Multiplexer1/1 -> FIR Compiler 7.4/1, FIR Compiler 7.3/1
  FIR Compiler 7.3/1 -> Terminator18/1
  Time Division Demultiplexer3/1 -> Delay8/1
  FIR Compiler 7.4/1 -> Terminator19/1
  FIR Compiler 7.3/5 -> Terminator15/1
  Delay8/1 -> AddSub3/1
  FIR Compiler 7.3/6 -> Terminator10/1
  Counter2/1 -> FIR Compiler 7.4/4, FIR Compiler 7.3/4, Relational4/2
  Delay4/1 -> AddSub2/1
  FIR Compiler 7.3/3 -> Terminator16/1
  FIR Compiler 7.4/5 -> Terminator13/1
  FIR Compiler 7.3/2 -> Terminator17/1
  m_axis_tdata1/1 -> Input/1
  FIR Compiler 7.4/4 -> Time Division Demultiplexer3/1
  Relational4/1 -> FIR Compiler 7.4/3, FIR Compiler 7.3/3
  FIR Compiler 7.4/2 -> Terminator20/1
  Time Division Demultiplexer3/2 -> AddSub3/2
  Time Division Demultiplexer2/2 -> AddSub2/2
  Constant12/1 -> Relational7/1
  FIR Compiler 7.6/3 -> Terminator32/1
  FIR Compiler 7.5/4 -> Time Division Demultiplexer4/1
  Time Division Demultiplexer4/1 -> Delay9/1
  FIR Compiler 7.6/6 -> Terminator25/1
  Time Division Multiplexer2/1 -> FIR Compiler 7.6/1, FIR Compiler 7.5/1
  FIR Compiler 7.5/1 -> Terminator29/1
  Time Division Demultiplexer5/1 -> Delay15/1
  FIR Compiler 7.6/1 -> Terminator30/1
  FIR Compiler 7.5/5 -> Terminator26/1
  Delay15/1 -> AddSub5/1
  FIR Compiler 7.5/6 -> Terminator23/1
  Counter4/1 -> FIR Compiler 7.6/4, FIR Compiler 7.5/4, Relational7/2
  Delay9/1 -> AddSub4/1
  FIR Compiler 7.5/3 -> Terminator27/1
  FIR Compiler 7.6/5 -> Terminator24/1
  FIR Compiler 7.5/2 -> Terminator28/1
  m_axis_tdata2/1 -> Input1/1
  FIR Compiler 7.6/4 -> Time Division Demultiplexer5/1
  Relational7/1 -> FIR Compiler 7.6/3, FIR Compiler 7.5/3
  FIR Compiler 7.6/2 -> Terminator31/1
  Time Division Demultiplexer5/2 -> AddSub5/2
  Time Division Demultiplexer4/2 -> AddSub4/2
  Constant16/1 -> Relational10/1
  FIR Compiler 7.8/3 -> Terminator43/1
  FIR Compiler 7.7/4 -> Time Division Demultiplexer6/1
  Time Division Demultiplexer6/1 -> Delay16/1
  FIR Compiler 7.8/6 -> Terminator36/1
  Time Division Multiplexer3/1 -> FIR Compiler 7.8/1, FIR Compiler 7.7/1
  FIR Compiler 7.7/1 -> Terminator40/1
  Time Division Demultiplexer7/1 -> Delay20/1
  FIR Compiler 7.8/1 -> Terminator41/1
  FIR Compiler 7.7/5 -> Terminator37/1
  Delay20/1 -> AddSub7/1
  FIR Compiler 7.7/6 -> Terminator34/1
  Counter6/1 -> FIR Compiler 7.8/4, FIR Compiler 7.7/4, Relational10/2
  FIR Compiler 7.7/3 -> Terminator38/1
  FIR Compiler 7.8/5 -> Terminator35/1
  FIR Compiler 7.7/2 -> Terminator39/1
  m_axis_tdata3/1 -> Input2/1
  FIR Compiler 7.8/4 -> Time Division Demultiplexer7/1
  Relational10/1 -> FIR Compiler 7.8/3, FIR Compiler 7.7/3
  AddSub7/1 -> m_axis_tdata8/1
  FIR Compiler 7.8/2 -> Terminator42/1
  Time Division Demultiplexer7/2 -> AddSub7/2
  s_axis_tvalid/1 -> m_axis_tvalid/1, FIR Compiler 7.7/2, FIR Compiler 7.6/2, FIR Compiler 7.5/2, FIR Compiler 7.4/2, FIR Compiler 7.2/2, FIR Compiler 7.1/2, FIR Compiler 7.3/2, FIR Compiler 7.8/2
  m_axis_tlast/1 -> m_tlast/1
  s_tvalid/1 -> s_axis_tvalid/1
  s_tlast/1 -> s_axis_tlast/1
  m_axis_tvalid/1 -> m_tvalid/1
  s_axis_tlast/1 -> m_axis_tlast/1
  AddSub/1 -> Gateway Out2/1, m_axis_tdata1/1
  AddSub1/1 -> m_axis_tdata2/1
  AddSub2/1 -> m_axis_tdata3/1
  m_axis_tdata4/1 -> Input3/1
  AddSub3/1 -> m_axis_tdata4/1
  m_axis_tdata5/1 -> Input4/1
  AddSub4/1 -> m_axis_tdata5/1
  m_axis_tdata6/1 -> Input5/1
  AddSub5/1 -> m_axis_tdata6/1
  m_axis_tdata7/1 -> Input6/1
  AddSub6/1 -> Gateway Out3/1, m_axis_tdata7/1
  m_axis_tdata8/1 -> Input7/1
  Gateway Out2/1 -> Time ScopeTwo/1
  Delay1/1 -> Gateway Out4/1, AddSub/1
  Time Division Demultiplexer/2 -> Gateway Out6/1, AddSub/2
  Time Division Demultiplexer/1 -> Delay1/1
  Gateway Out3/1 -> Time Scope3/1
  Gateway Out4/1 -> Time Scope4/1
  Gateway Out6/1 -> Time Scope6/1
  Gateway Out7/1 -> Time Scope7/1
  Delay16/1 -> Gateway Out7/1, AddSub6/1
  Gateway Out8/1 -> Time Scope8/1
  Time Division Demultiplexer6/2 -> Gateway Out8/1, AddSub6/2
  s_axis_tuser/1 -> m_axis_tuser/1
  m_axis_tuser/1 -> m_tuser/1
  s_tuser/1 -> s_axis_tuser/1

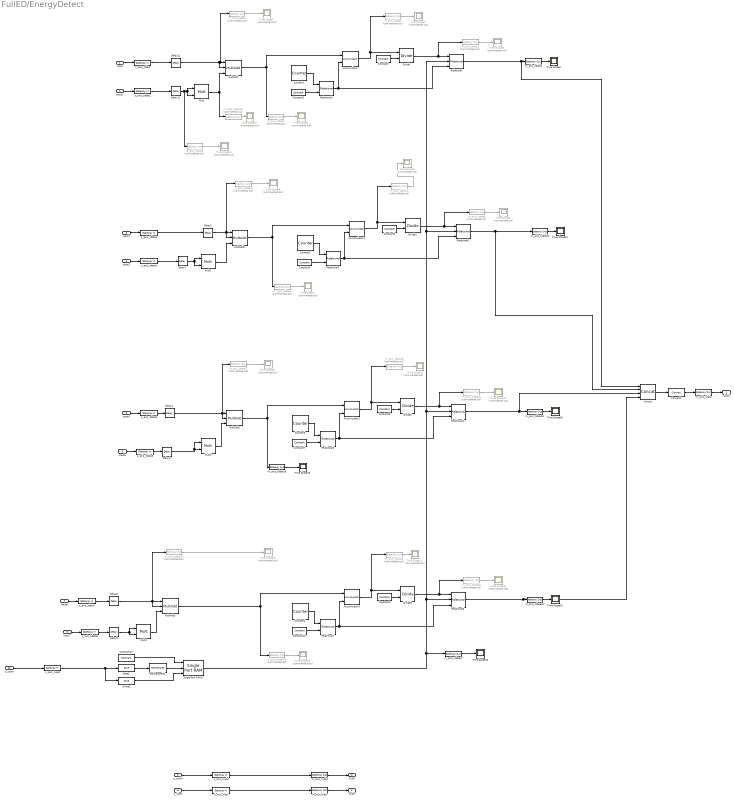
== system FullED/EnergyDetect ==
  Input : Inport
  Input1 : Inport  Port=2
  Input2 : Inport  Port=3
  Input3 : Inport  Port=4
  Input4 : Inport  Port=5
  Input5 : Inport  Port=6
  Input6 : Inport  Port=7
  Input7 : Inport  Port=8
  s_tvalid : Inport  Port=9
  s_tuser : Inport  Port=10
  s_tlast : Inport  Port=11
  Accumulator{,1..3} (4 alike) : hdlBasic/Accumulator  operation=Add  n_bits=64  overflow=Wrap  scale=1  rst=on  hasbypass=off  en=off  latency=1  msb_inp=100  msb=100  lsb=-100  use_behavioral_HDL=on  implementation=Fabric  XmcBlockStatus=1  maskContainerNames=group3  block_type=accum  block_config=sysgen:Accum_config  block_width=566  block_height=845
  Concat : hdlBasic/Concat  num_inputs=4  XmcBlockStatus=1  maskContainerNames=group1  block_type=concat  block_config=sysgen:Concat_config
  Constant{,1..3,6..7,9..10} (8 alike) : hdlBasic/Constant  const=512  gui_display_data_type=Fixed-point  arith_type=Unsigned  n_bits=16  bin_pt=0  preci_type=Single  exp_width=8  frac_width=24  explicit_period=off  period=1  XmcBlockStatus=1  maskContainerNames=tabcontainer1  block_type=constant  block_config=sysgen:Constant_config
  Constant11 : hdlBasic/Constant  const=1.0  gui_display_data_type=Fixed-point  arith_type=Unsigned  n_bits=1  bin_pt=0  preci_type=Single  exp_width=8  frac_width=24  explicit_period=off  period=1  XmcBlockStatus=1  maskContainerNames=tabcontainer1  block_type=constant  block_config=sysgen:Constant_config
  Convert1 : hdlBasic/Convert  gui_display_data_type=Fixed-point  arith_type=Signed (2's comp)  n_bits=32  bin_pt=16  float_type=Single  exp_bits=8  fraction_bits=24  quantization=Truncate  overflow=Wrap  en=off  latency=1  pipeline=off  XmcBlockStatus=1  maskContainerNames=group2  block_type=convert  block_config=sysgen:Convert_config  block_width=595  block_height=885
  Counter{1..4} (4 alike) : hdlBasic/Counter  cnt_type=Count limited  cnt_to=512  operation=Up  start_count=0  cnt_by_val=1  arith_type=Unsigned  n_bits=16  bin_pt=0  load_pin=off  rst=off  en=off  explicit_period=Explicit  period=1/fs  use_behavioral_HDL=off  implementation=Fabric  XmcBlockStatus=1  maskContainerNames=group1  block_type=counter  block_config=sysgen:Counter_config  block_width=531  block_height=1023
  Data3 : hdlBasic/Slice  nbits=15  boolean_output=off  mode=Upper Bit Location + Width  bit1=15  base1=LSB of Input  bit0=16*8-(16*1)  base0=LSB of Input  XmcBlockStatus=1  maskContainerNames=group1  block_type=slice  block_config=sysgen:Slice_config
  Delay{1,3,5,11} (4 alike) : hdlBasic/Delay  rst=off  en=off  latency=1  reg_retiming=off  XmcBlockStatus=1  maskContainerNames=group1  block_type=delay  block_config=sysgen:Delay_config
  Delay{2,4,6,12} (4 alike) : hdlBasic/Delay  rst=off  en=off  latency=4  reg_retiming=off  XmcBlockStatus=1  maskContainerNames=group1  block_type=delay  block_config=sysgen:Delay_config
  Divide{,1..3} (4 alike) : hdlBasic/Divide  flow_control=NonBlocking  axi_optimize_goal=Resources  algorithm_type=Radix2  fractional_width=16  latency=1  rate=1  has_a_tlast=off  has_a_tuser=off  has_b_tlast=off  has_b_tuser=off  en=off  has_result_tready=off  result_tlast_behv=Pass_A_TLAST  has_underflow=off  has_overflow=off  has_invalid_op=off  has_divide_by_zero=off  fpo_op_type=mergeddivide  XmcBlockStatus=1  maskContainerNames=tabcontainer1  block_type=divide  block_config=sysgen:FPOBlockDescriptor_config
  Mult{,1..3} (4 alike) : hdlBasic/Mult  precision=User Defined  arith_type="Signed  (2's comp)"  n_bits=32  bin_pt=28  quantization=Truncate  overflow=Wrap  en=off  latency=3  use_behavioral_HDL=off  opt=Speed  use_embedded=on  optimum_pipeline=off  pipeline=on  use_rpm=on  placement_style=Triangular  XmcBlockStatus=1  maskContainerNames=group1  block_type=mult  block_config=sysgen:Mult_config  block_width=598  block_height=876
  MultAdd{,1..3} (4 alike) : hdlBasic/MultAdd  mode=Addition  en=off  latency=0  precision=User Defined  arith_type=Unsigned  n_bits=48  bin_pt=40  XmcBlockStatus=1  maskContainerNames=tabcontainer1  block_type=multadd  block_config=sysgen:MultAdd_config
  Reinterpret11 : hdlBasic/Reinterpret  force_arith_type=on  arith_type=Unsigned  force_bin_pt=on  bin_pt=10  XmcBlockStatus=1  maskContainerNames=group1  block_type=reinterpret  block_config=sysgen:Reinterpret_config
  Relational{,1,4,6} (4 alike) : hdlBasic/Relational  mode=a>b  op_type=Bool  en=on  latency=1  XmcBlockStatus=1  maskContainerNames=tabcontainer1  block_type=relational  block_config=sysgen:Relational_config
  Relational{2..3,5,7} (4 alike) : hdlBasic/Relational  mode=a=b  op_type=Bool  en=off  latency=1  XmcBlockStatus=1  maskContainerNames=tabcontainer1  block_type=relational  block_config=sysgen:Relational_config
  Single Port RAM3 : hdlBasic/Single Port RAM  depth=2  initVector=[0 0]  distributed_mem=Distributed memory  write_mode=Read After Write  rst=off  init_reg=0  en=off  optimize_latency=on  latency=1  optimize=Area  dbl_ovrd=off  simulation_type=fast_sim  XmcBlockStatus=1  maskContainerNames=tabcontainer1  block_type=spram  block_config=sysgen:SPRAM_config
  Time Scope{1..3,5..9,11..12,14..15,17..21} (17 alike) : Scope  Commented=on
  Time Scope{4,10,13,16,22..23} (6 alike) : Scope
  Write3 : hdlBasic/Slice  nbits=1  boolean_output=on  mode=Upper Bit Location + Width  bit1=0  base1=LSB of Input  bit0=16*8-(16*1)  base0=LSB of Input  XmcBlockStatus=1  maskContainerNames=group1  block_type=slice  block_config=sysgen:Slice_config
  m_axis_tdata : hdlBasic/Gateway Out  inherit_from_input=on  hdl_port=on  rows=1  columns=1  UseAsDAC=off  DACChannel='1'  interface=None  automatic_assignment=on  address_offset=hex2dec('00')  intf_name=''  intf_description=''  timing_constraint=None  locs_specified=off  LOCs={}  io_standard={}  XmcBlockStatus=1  maskContainerNames=group4  block_type=gatewayout  block_config=sysgen:gateway_out_config  block_width_w=590  block_height_w=620  block_width=620  block_height=750
  m_axis_tdata{1..4,6,8..11,13,15,17..18,22..25} (17 alike) : hdlBasic/Gateway Out  Commented=on  inherit_from_input=on  hdl_port=off  rows=1  columns=1  UseAsDAC=off  DACChannel='1'  interface=None  automatic_assignment=on  address_offset=hex2dec('00')  intf_name=''  intf_description=''  timing_constraint=None  locs_specified=off  LOCs={}  io_standard={}  XmcBlockStatus=1  maskContainerNames=group4  block_type=gatewayout  block_config=sysgen:gateway_out_config  block_width_w=590  block_height_w=620  block_width=620  block_height=750
  m_axis_tdata{5,12,16,19,26..27} (6 alike) : hdlBasic/Gateway Out  inherit_from_input=on  hdl_port=off  rows=1  columns=1  UseAsDAC=off  DACChannel='1'  interface=None  automatic_assignment=on  address_offset=hex2dec('00')  intf_name=''  intf_description=''  timing_constraint=None  locs_specified=off  LOCs={}  io_standard={}  XmcBlockStatus=1  maskContainerNames=group4  block_type=gatewayout  block_config=sysgen:gateway_out_config  block_width_w=590  block_height_w=620  block_width=620  block_height=750
  m_axis_tlast : hdlBasic/Gateway Out  inherit_from_input=on  hdl_port=on  rows=1  columns=1  UseAsDAC=off  DACChannel='1'  interface=None  automatic_assignment=on  address_offset=hex2dec('00')  intf_name=''  intf_description=''  timing_constraint=None  locs_specified=off  LOCs={}  io_standard={}  XmcBlockStatus=1  maskContainerNames=group4  block_type=gatewayout  block_config=sysgen:gateway_out_config  block_width_w=590  block_height_w=620  block_width=620  block_height=750
  m_axis_tvalid : hdlBasic/Gateway Out  inherit_from_input=on  hdl_port=on  rows=1  columns=1  UseAsDAC=off  DACChannel='1'  interface=None  automatic_assignment=on  address_offset=hex2dec('00')  intf_name=''  intf_description=''  timing_constraint=None  locs_specified=off  LOCs={}  io_standard={}  XmcBlockStatus=1  maskContainerNames=group4  block_type=gatewayout  block_config=sysgen:gateway_out_config  block_width_w=590  block_height_w=620  block_width=620  block_height=750
  s_axis_tdata{,2..8} (8 alike) : hdlBasic/Gateway In  gui_display_data_type=Fixed-point  arith_type=Signed (2's comp)  n_bits=16  bin_pt=14  preci_type=Single  exp_width=8  frac_width=24  rows=1  columns=1  quantization="Round  (unbiased: +/- Inf)"  overflow=Saturate  period=1/fs  UseAsADC=off  ADCChannel='1'  interface=None  automatic_assignment=on  address_offset=hex2dec('00')  intf_name=''  intf_description=''  default_value=0  timing_constraint=None  locs_specified=off  LOCs={}  io_standard={}  inherit_from_input=off  hdl_port=on  XmcBlockStatus=1  maskContainerNames=group4  block_type=gatewayin  block_config=sysgen:gateway_in_config  block_width_w=590  block_height_w=620  block_width=640  block_height=850
  s_axis_tlast : hdlBasic/Gateway In  gui_display_data_type=Boolean  arith_type=Boolean  n_bits=16  bin_pt=14  preci_type=Single  exp_width=8  frac_width=24  rows=1  columns=1  quantization="Round  (unbiased: +/- Inf)"  overflow=Saturate  period=1/fs  UseAsADC=off  ADCChannel='1'  interface=None  automatic_assignment=on  address_offset=hex2dec('00')  intf_name=''  intf_description=''  default_value=0  timing_constraint=None  locs_specified=off  LOCs={}  io_standard={}  inherit_from_input=off  hdl_port=on  XmcBlockStatus=1  maskContainerNames=group4  block_type=gatewayin  block_config=sysgen:gateway_in_config  block_width_w=590  block_height_w=620  block_width=640  block_height=850
  s_axis_tuser : hdlBasic/Gateway In  gui_display_data_type=Fixed-point  arith_type=Unsigned  n_bits=32  bin_pt=0  preci_type=Single  exp_width=8  frac_width=24  rows=1  columns=1  quantization="Round  (unbiased: +/- Inf)"  overflow=Saturate  period=1/fs  UseAsADC=off  ADCChannel='1'  interface=None  automatic_assignment=on  address_offset=hex2dec('00')  intf_name=''  intf_description=''  default_value=0  timing_constraint=None  locs_specified=off  LOCs={}  io_standard={}  inherit_from_input=off  hdl_port=on  XmcBlockStatus=1  maskContainerNames=group4  block_type=gatewayin  block_config=sysgen:gateway_in_config  block_width_w=590  block_height_w=620  block_width=640  block_height=850
  s_axis_tvalid : hdlBasic/Gateway In  gui_display_data_type=Boolean  arith_type=Boolean  n_bits=16  bin_pt=14  preci_type=Single  exp_width=8  frac_width=24  rows=1  columns=1  quantization="Round  (unbiased: +/- Inf)"  overflow=Saturate  period=1/fs  UseAsADC=off  ADCChannel='1'  interface=None  automatic_assignment=on  address_offset=hex2dec('00')  intf_name=''  intf_description=''  default_value=0  timing_constraint=None  locs_specified=off  LOCs={}  io_standard={}  inherit_from_input=off  hdl_port=on  XmcBlockStatus=1  maskContainerNames=group4  block_type=gatewayin  block_config=sysgen:gateway_in_config  block_width_w=590  block_height_w=620  block_width=640  block_height=850
  Out1 : Outport
  Out5 : Outport  Port=2
  Out6 : Outport  Port=3
  wires:
  s_axis_tuser/1 -> Write3/1, Data3/1
  m_axis_tdata25/1 -> Time Scope21/1
  Relational4/1 -> Concat/3, m_axis_tdata19/1
  Divide2/1 -> m_axis_tdata15/1, Relational4/1
  Delay1/1 -> Mult1/2, Mult1/1
  s_axis_tlast/1 -> m_axis_tlast/1
  Accumulator2/1 -> m_axis_tdata18/1, Divide2/1
  Counter1/1 -> Relational2/1
  Divide/1 -> m_axis_tdata1/1, Relational/1
  Single Port RAM3/1 -> m_axis_tdata27/1, Relational/2, Relational1/2, Relational4/2, Relational6/2
  Relational5/1 -> Accumulator2/2, Relational4/3
  m_axis_tdata9/1 -> Time Scope7/1
  Constant6/1 -> Divide2/2
  Write3/1 -> Single Port RAM3/3
  Relational/1 -> Concat/1, m_axis_tdata5/1
  m_axis_tdata18/1 -> Time Scope15/1
  MultAdd2/1 -> Accumulator2/1, m_axis_tdata16/1
  m_axis_tdata3/1 -> Time Scope2/1
  MultAdd1/1 -> Accumulator1/1, m_axis_tdata9/1
  m_axis_tdata15/1 -> Time Scope12/1
  Constant11/1 -> Single Port RAM3/1
  Accumulator1/1 -> m_axis_tdata11/1, Divide1/1
  Delay2/1 -> MultAdd1/2, m_axis_tdata10/1, MultAdd1/1
  Counter2/1 -> Relational3/1
  Counter3/1 -> Relational5/1
  Constant7/1 -> Relational5/2
  m_axis_tdata17/1 -> Time Scope14/1
  m_axis_tdata27/1 -> Time Scope23/1
  Divide1/1 -> m_axis_tdata8/1, Relational1/1
  Relational3/1 -> Accumulator1/2, Relational1/3
  s_axis_tdata3/1 -> Delay2/1
  Accumulator/1 -> m_axis_tdata4/1, Divide/1
  Divide3/1 -> m_axis_tdata22/1, Relational6/1
  Delay12/1 -> MultAdd/2, m_axis_tdata3/1, MultAdd/1
  m_axis_tdata19/1 -> Time Scope16/1
  m_axis_tdata16/1 -> Time Scope13/1
  Mult2/1 -> MultAdd2/3
  s_axis_tdata2/1 -> Delay11/1
  Constant/1 -> Divide/2
  s_tuser/1 -> s_axis_tuser/1
  MultAdd/1 -> Accumulator/1, m_axis_tdata2/1
  s_tvalid/1 -> s_axis_tvalid/1
  s_axis_tdata/1 -> Delay12/1
  Constant2/1 -> Relational2/2
  m_axis_tdata12/1 -> Time Scope10/1
  m_axis_tdata1/1 -> Time Scope5/1
  m_axis_tdata2/1 -> Time Scope1/1
  m_axis_tdata5/1 -> Time Scope4/1
  Relational7/1 -> Accumulator3/2, Relational6/3
  Accumulator3/1 -> m_axis_tdata25/1, Divide3/1
  Counter4/1 -> Relational7/1
  m_axis_tdata24/1 -> Time Scope20/1
  Constant9/1 -> Divide3/2
  m_axis_tdata22/1 -> Time Scope18/1
  Constant10/1 -> Relational7/2
  m_axis_tdata23/1 -> Time Scope19/1
  m_axis_tdata4/1 -> Time Scope3/1
  Data3/1 -> Reinterpret11/1
  m_axis_tdata26/1 -> Time Scope22/1
  Reinterpret11/1 -> Single Port RAM3/2
  Mult3/1 -> MultAdd3/3
  Relational2/1 -> Accumulator/2, Relational/3
  m_axis_tdata11/1 -> Time Scope9/1
  m_axis_tdata10/1 -> Time Scope8/1
  Constant1/1 -> Divide1/2
  m_axis_tdata8/1 -> Time Scope6/1
  Relational1/1 -> Concat/2, m_axis_tdata12/1
  s_axis_tdata4/1 -> Delay1/1
  Constant3/1 -> Relational3/2
  Mult1/1 -> MultAdd1/3
  s_axis_tvalid/1 -> m_axis_tvalid/1
  s_tlast/1 -> s_axis_tlast/1
  m_axis_tvalid/1 -> Out5/1
  m_axis_tlast/1 -> Out6/1
  Delay6/1 -> m_axis_tdata24/1, MultAdd3/2, MultAdd3/1
  Delay5/1 -> Mult3/1, Mult3/2
  Delay4/1 -> MultAdd2/2, m_axis_tdata17/1, MultAdd2/1
  Delay3/1 -> Mult2/1, Mult2/2
  Input/1 -> s_axis_tdata/1
  Input1/1 -> s_axis_tdata2/1
  Input2/1 -> s_axis_tdata3/1
  Input3/1 -> s_axis_tdata4/1
  Input4/1 -> s_axis_tdata5/1
  s_axis_tdata5/1 -> Delay4/1
  Input5/1 -> s_axis_tdata6/1
  Input6/1 -> s_axis_tdata7/1
  s_axis_tdata7/1 -> Delay6/1
  Input7/1 -> s_axis_tdata8/1
  s_axis_tdata8/1 -> Delay5/1
  s_axis_tdata6/1 -> Delay3/1
  Delay11/1 -> m_axis_tdata6/1, Mult/2, Mult/1
  m_axis_tdata6/1 -> Time Scope11/1
  Mult/1 -> MultAdd/3, m_axis_tdata13/1
  m_axis_tdata13/1 -> Time Scope17/1
  MultAdd3/1 -> m_axis_tdata23/1, Accumulator3/1
  Relational6/1 -> Concat/4, m_axis_tdata26/1
  m_axis_tdata/1 -> Out1/1
  Convert1/1 -> m_axis_tdata/1
  Concat/1 -> Convert1/1
